simulink model "Hw3_ME8352sim"  (R2020b)
settings: Solver=VariableStepAuto  StartTime=0.0  StopTime=t_sim  RelTol=1e-6
values from neighbouring files (symbols this model uses):
  K_ = K_array(i)    [Hw3_ME8352.m]
  x_0 = x0_array(ii)    [Hw3_ME8352.m]
  xdot_0 = xdot0_array(iii)    [Hw3_ME8352.m]
settings Model: Creator=dempseca  LastModifiedBy=dempseca

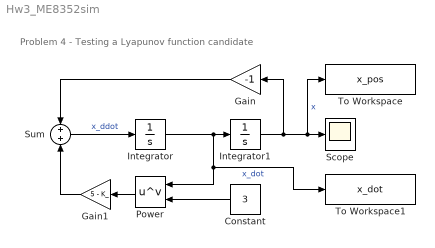
== system Hw3_ME8352sim ==
  note: Problem 4 - Testing a Lyapunov function candidate
  Constant : Constant  Value=3
  Gain : Gain  Gain=-1
  Gain1 : Gain  Gain=5 - K_
  Integrator : Integrator  InitialCondition=xdot_0  LimitOutput=on  UpperSaturationLimit=100  LowerSaturationLimit=-100
  Integrator1 : Integrator  InitialCondition=x_0  LimitOutput=on  UpperSaturationLimit=100  LowerSaturationLimit=-100
  Power : Math  Operator=pow  SaturateOnIntegerOverflow=on
  Scope : Scope
  Sum : Sum
  To Workspace : ToWorkspace  VariableName=x_pos  SaveFormat=Timeseries  SampleTime=-1
  To Workspace1 : ToWorkspace  VariableName=x_dot  SaveFormat=Timeseries  SampleTime=-1
  wires:
  Integrator/1 -> To Workspace1/1, Power/1, Integrator1/1  "x_dot"
  Integrator1/1 -> Gain/1, To Workspace/1, Scope/1  "x"
  Sum/1 -> Integrator/1  "x_ddot"
  Gain/1 -> Sum/1
  Gain1/1 -> Sum/2
  Power/1 -> Gain1/1
  Constant/1 -> Power/2
